simulink model "uas_sim"  (R2020b)
settings: Solver=VariableStepAuto  StartTime=0.0  StopTime=10.0  RelTol=1e-3  SampleTimeConstraint=STIndependent
values from neighbouring files (symbols this model uses):
  framePeriod_s = 1/frameRate_hz    (= 0.02)    [autocode_setup.m]
undefined symbols (not defined in the file or in its folder): Aircraft, datetime, datevec, Earth, Env, InitCond, Telem, WGS84
libraries: aerolibconvert2 x8, simulink x8, aerolibadyn x3, aerolibasang x3, aerolibtransform2 x2, aerolibgravity2 x2, aerolibatmos2 x1, sharedutil x1, aerolibbdyn x1, shared6dof x1
(part 2 of 2)

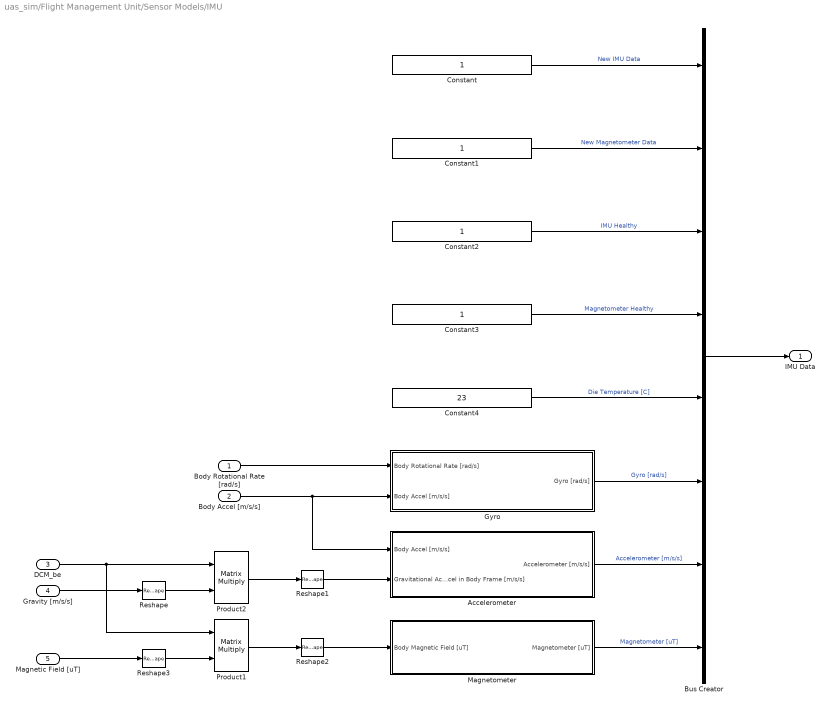
== system uas_sim/Flight Management Unit/Sensor Models/IMU ==
  Body Rotational Rate [rad/s] : Inport
  Body Accel [m/s/s] : Inport  Port=2
  DCM_be : Inport  Port=3
  Gravity [m/s/s] : Inport  Port=4
  Magnetic Field [uT] : Inport  Port=5
  Accelerometer : Subsystem
  Bus Creator : BusCreator  Inputs=8
  Constant{,1..3} (4 alike) : Constant
  Constant4 : Constant  Value=23
  Gyro : Subsystem
  Magnetometer : Subsystem
  Product1 : Product  Multiplication=Matrix(*)
  Product2 : Product  Multiplication=Matrix(*)
  Reshape : Reshape  OutputDimensionality=Column vector (2-D)
  Reshape1 : Reshape
  Reshape2 : Reshape
  Reshape3 : Reshape  OutputDimensionality=Column vector (2-D)
  IMU Data : Outport
  wires:
  Body Accel [m/s/s]/1 -> Accelerometer/1(Body Accel [m/s/s]), Gyro/2(Body Accel [m/s/s])
  DCM_be/1 -> Product2/1, Product1/1
  Gravity [m/s/s]/1 -> Reshape/1
  Bus Creator/1 -> IMU Data/1
  Product2/1 -> Reshape1/1
  Reshape1/1 -> Accelerometer/2(Gravitational Accel in Body Frame [m/s/s])
  Body Rotational Rate [rad/s]/1 -> Gyro/1(Body Rotational Rate [rad/s])
  Reshape2/1 -> Magnetometer/1(Body Magnetic Field [uT])
  Product1/1 -> Reshape2/1
  Reshape3/1 -> Product1/2
  Magnetic Field [uT]/1 -> Reshape3/1
  Magnetometer/1(Magnetometer [uT]) -> Bus Creator/8  "Magnetometer [uT]"
  Accelerometer/1(Accelerometer [m/s/s]) -> Bus Creator/7  "Accelerometer [m/s/s]"
  Gyro/1(Gyro [rad/s]) -> Bus Creator/6  "Gyro [rad/s]"
  Reshape/1 -> Product2/2
  Constant1/1 -> Bus Creator/2  "New Magnetometer Data"
  Constant/1 -> Bus Creator/1  "New IMU Data"
  Constant2/1 -> Bus Creator/3  "IMU Healthy"
  Constant3/1 -> Bus Creator/4  "Magnetometer Healthy"
  Constant4/1 -> Bus Creator/5  "Die Temperature [C]"

== system uas_sim/Flight Management Unit/Sensor Models/Static Pressure Sensor ==
  Pressure : Inport
  Add : Sum  Inputs=+++
  Band-Limited White Noise : simulink/Sources/Band-Limited White Noise  Cov=Aircraft.Sensors.StaticPres.noise_pa  Ts=0.1  seed=[23341]
  Bus Creator : BusCreator  Inputs=4
  Constant : Constant  Value=Aircraft.Sensors.StaticPres.bias_pa
  Constant1 : Constant  Value=Aircraft.Sensors.StaticPres.scale_factor
  Constant2 : Constant  Value=23
  Constant3 : Constant
  Constant4 : Constant
  Product : Product
  Saturation : Saturate  UpperLimit=Aircraft.Sensors.StaticPres.upper_limit_pa  LowerLimit=Aircraft.Sensors.StaticPres.lower_limit_pa
  Pressure Data : Outport
  wires:
  Constant4/1 -> Bus Creator/1  "New Data"
  Constant3/1 -> Bus Creator/2  "Healthy"
  Constant2/1 -> Bus Creator/4  "Die Temperature [C]"
  Saturation/1 -> Bus Creator/3  "Pressure [Pa]"
  Band-Limited White Noise/1 -> Add/1
  Constant/1 -> Add/2
  Add/1 -> Saturation/1
  Product/1 -> Add/3
  Pressure/1 -> Product/1
  Constant1/1 -> Product/2
  Bus Creator/1 -> Pressure Data/1

== system uas_sim/Vehicle/Forces and Moments/Aerodynamic ==
  note: C6 = [CD, CY, CLift, CL, CM, CN]
  Body Velocity [m/s] : Inport
  Body Rotational Rates [rad/s] : Inport  Port=2
  Surface Positions [rad] : Inport  Port=3
  Dynamic Pressure [Pa] : Inport  Port=4
  Angle of Attack [rad] : Inport  Port=5
  Sideslip Angle [rad] : Inport  Port=6
  Airspeed [m/s] : Inport  Port=7
  Add : Sum  Inputs=+++
  Aerodynamic Forces and Moments Coef Axis Variant : Subsystem  Variant=on
  Base Airframe : Subsystem
  Control Derivatives : Subsystem
  Dynamic Derivatives : Subsystem
  Fxyz Mxzy : Outport
  wires:
  Base Airframe/1(C6) -> Add/1
  Dynamic Derivatives/1(dC6) -> Add/2
  Sideslip Angle [rad]/1 -> Base Airframe/2(Sideslip Angle [rad])
  Angle of Attack [rad]/1 -> Base Airframe/1(Angle of Attack [rad]), Control Derivatives/2(Angle of Attack [rad]), Dynamic Derivatives/3(Angle of Attack [rad])
  Body Rotational Rates [rad/s]/1 -> Dynamic Derivatives/2(Body Rotational Rate [rad/s])
  Airspeed [m/s]/1 -> Dynamic Derivatives/1(Airspeed [m/s])
  Surface Positions [rad]/1 -> Control Derivatives/1(Surface Positions [rad])
  Control Derivatives/1(dC6) -> Add/3
  Add/1 -> Aerodynamic Forces and Moments Coef Axis Variant/1(Coef)
  Body Velocity [m/s]/1 -> Aerodynamic Forces and Moments Coef Axis Variant/3(Body Velocity [m/s])
  Dynamic Pressure [Pa]/1 -> Aerodynamic Forces and Moments Coef Axis Variant/2(Dynamic Pressure [Pa])
  Aerodynamic Forces and Moments Coef Axis Variant/1(Fxyz Mxyz) -> Fxyz Mxzy/1

== system uas_sim/Vehicle/Forces and Moments/Gravitational ==
  Gravity [m/s/s] : Inport
  DCM_be : Inport  Port=2
  Gravity Moment : Constant  Value=[0 0 0]
  Mux : Mux  Inputs=2
  Product : Product
  Product1 : Product  Multiplication=Matrix(*)
  Reshape : Reshape  OutputDimensionality=Column vector (2-D)
  Reshape1 : Reshape
  UAV Mass : Constant  Value=Aircraft.Mass.mass_kg
  Fxyz Mxyz : Outport
  wires:
  UAV Mass/1 -> Product/2
  Product/1 -> Product1/2  "Gravity Force NED [N]"
  DCM_be/1 -> Product1/1
  Gravity Moment/1 -> Mux/2
  Mux/1 -> Fxyz Mxyz/1
  Reshape/1 -> Product/1
  Gravity [m/s/s]/1 -> Reshape/1
  Reshape1/1 -> Mux/1
  Product1/1 -> Reshape1/1  "Gravity Force Body [N]"

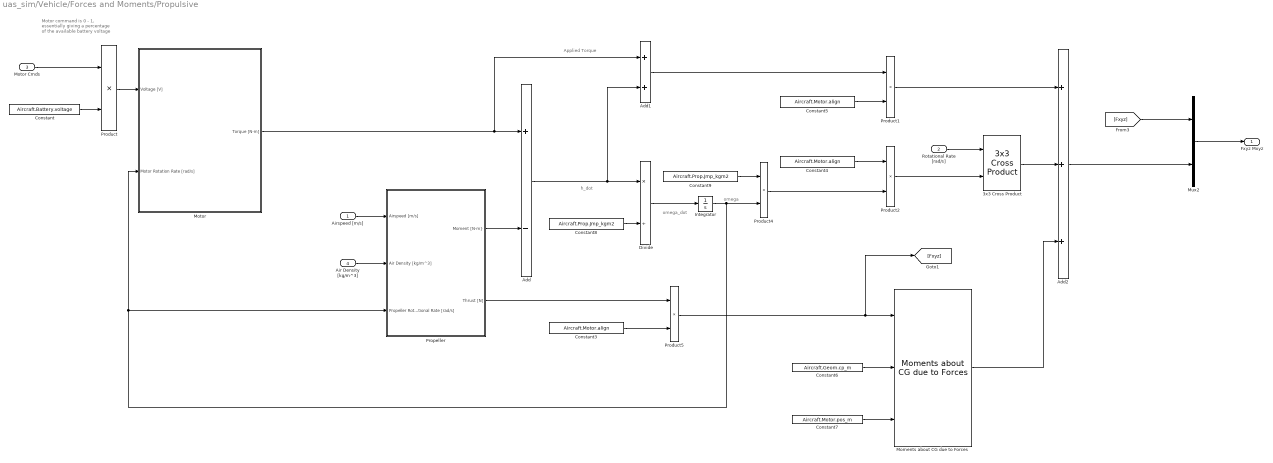
== system uas_sim/Vehicle/Forces and Moments/Propulsive ==
  note: Applied Torque
  note: omega_dot
  note: Motor command is 0 - 1,
      | essentially giving a percentage
      | of the available battery voltage
  note: h_dot
  note: omega
  Airspeed [m/s] : Inport
  Rotational Rate [rad/s] : Inport  Port=2
  Motor Cmds : Inport  Port=3
  Air Density [kg/m^3] : Inport  Port=4
  3x3 Cross Product : sharedutil/3x3 Cross Product  aMode=aMode
      settings: SourceProductBaseCode=AE,PW,MT,UV,VE,VP
  Add : Sum  Inputs=+-
  Add1 : Sum
  Add2 : Sum  Inputs=+++
  Constant : Constant  Value=Aircraft.Battery.voltage
  Constant3 : Constant  Value=Aircraft.Motor.align
  Constant4 : Constant  Value=Aircraft.Motor.align
  Constant5 : Constant  Value=Aircraft.Motor.align
  Constant6 : Constant  Value=Aircraft.Geom.cp_m
  Constant7 : Constant  Value=Aircraft.Motor.pos_m
  Constant8 : Constant  Value=Aircraft.Prop.Jmp_kgm2
  Constant9 : Constant  Value=Aircraft.Prop.Jmp_kgm2
  Divide : Product  Inputs=*/
  Integrator : Integrator  InitialCondition=InitCond.engine_speed_radps  LowerSaturationLimit=1
  Moments about CG due to Forces : aerolibbdyn/Moments about CG  due to Forces
      settings: SourceProductBaseCode=AE
  Motor : Subsystem
  Mux2 : Mux  Inputs=2
  Product{,1..2,4..5} (5 alike) : Product
  Propeller : Subsystem
  Fxyz Mxyz : Outport
  wires:
  Integrator/1 -> Product4/2, Propeller/3(Propeller Rotational Rate [rad/s]), Motor/2(Motor Rotation Rate [rad/s])
  [Fxyz] -> Mux2/1
  Constant4/1 -> Product2/1
  Motor/1(Torque [N-m]) -> Add1/1, Add/1
  Add1/1 -> Product1/1
  Product/1 -> Motor/1(Voltage [V])
  Moments about CG due to Forces/1 -> Add2/3
  Product1/1 -> Add2/1
  Add2/1 -> Mux2/2
  Constant9/1 -> Product4/1
  Propeller/2(Thrust [N]) -> Product5/1
  3x3 Cross Product/1 -> Add2/2
  Mux2/1 -> Fxyz Mxyz/1
  Constant/1 -> Product/2
  Product5/1 -> [Fxyz], Moments about CG due to Forces/1
  Constant3/1 -> Product5/2
  Divide/1 -> Integrator/1
  Add/1 -> Add1/2, Divide/1
  Propeller/1("Moment [N-m}") -> Add/2
  Constant6/1 -> Moments about CG due to Forces/2
  Rotational Rate [rad/s]/1 -> 3x3 Cross Product/1
  Air Density [kg/m^3]/1 -> Propeller/2(Air Density [kg/m^3])
  Product4/1 -> Product2/2
  Constant7/1 -> Moments about CG due to Forces/3
  Constant8/1 -> Divide/2
  Product2/1 -> 3x3 Cross Product/2
  Constant5/1 -> Product1/2
  Motor Cmds/1 -> Product/1
  Airspeed [m/s]/1 -> Propeller/1(Airspeed [m/s])

== system uas_sim/Vehicle/Vehicle Model/Norm ==
  2D Vector : Inport
  Product : Product
  Sqrt : Sqrt  SaturateOnIntegerOverflow=on
  Sum of Elements : Sum  Inputs=+
  Norm : Outport
  wires:
  2D Vector/1 -> Product/2, Product/1
  Product/1 -> Sum of Elements/1
  Sum of Elements/1 -> Sqrt/1
  Sqrt/1 -> Norm/1

== system uas_sim/Flight Management Unit/Control Laws/Virtual to Non-Virtual Mapping1/Virtual to Non-Virtual Mapping1 ==
  Virtual : Inport
  Bus Creator : BusCreator  Inputs=10
  Bus Selector : BusSelector  OutputSignals=New Data,Lost Frame,Failsafe,Throttle Enable,Mode 0,Mode 1,Throttle,Pitch,Roll,Yaw
  Data Type Conversion{,1..3} (4 alike) : DataTypeConversion  OutDataTypeStr=boolean
  Data Type Conversion4 : DataTypeConversion  OutDataTypeStr=int8
  Data Type Conversion5 : DataTypeConversion  OutDataTypeStr=int8
  Data Type Conversion{6..9} (4 alike) : DataTypeConversion  OutDataTypeStr=single
  Non-Virtual : Outport  OutDataTypeStr=Bus: InceptorData
  wires:
  Virtual/1 -> Bus Selector/1
  Bus Creator/1 -> Non-Virtual/1
  Bus Selector/1 -> Data Type Conversion/1  "<New Data>"
  Data Type Conversion/1 -> Bus Creator/1  "new_data"
  Bus Selector/2 -> Data Type Conversion1/1  "<Lost Frame>"
  Bus Selector/3 -> Data Type Conversion2/1  "<Failsafe>"
  Bus Selector/4 -> Data Type Conversion3/1  "<Throttle Enable>"
  Bus Selector/5 -> Data Type Conversion4/1  "<Mode 0>"
  Bus Selector/6 -> Data Type Conversion5/1  "<Mode 1>"
  Bus Selector/7 -> Data Type Conversion6/1  "<Throttle>"
  Bus Selector/8 -> Data Type Conversion7/1  "<Pitch>"
  Bus Selector/9 -> Data Type Conversion8/1  "<Roll>"
  Bus Selector/10 -> Data Type Conversion9/1  "<Yaw>"
  Data Type Conversion1/1 -> Bus Creator/2  "lost_frame"
  Data Type Conversion2/1 -> Bus Creator/3  "failsafe"
  Data Type Conversion3/1 -> Bus Creator/4  "throttle_en"
  Data Type Conversion4/1 -> Bus Creator/5  "mode0"
  Data Type Conversion5/1 -> Bus Creator/6  "mode1"
  Data Type Conversion6/1 -> Bus Creator/7  "throttle"
  Data Type Conversion7/1 -> Bus Creator/8  "pitch"
  Data Type Conversion8/1 -> Bus Creator/9  "roll"
  Data Type Conversion9/1 -> Bus Creator/10  "yaw"

== system uas_sim/Flight Management Unit/Control Laws/Virtual to Non-Virtual Mapping1/Virtual to Non-Virtual Mapping2 ==
  Virtual : Inport
  Bus Creator : BusCreator  Inputs=8
  Bus Selector : BusSelector  OutputSignals=New IMU Data,New Magnetometer Data,IMU Healthy,Magnetometer Healthy,Die Temperature [C],Accelerometer [m/s/s],Gyro [rad/s],Magnetometer [uT]
  Data Type Conversion{,1..3} (4 alike) : DataTypeConversion  OutDataTypeStr=boolean
  Data Type Conversion{4..7} (4 alike) : DataTypeConversion  OutDataTypeStr=single
  Non-Virtual : Outport  OutDataTypeStr=Bus: ImuData
  wires:
  Bus Creator/1 -> Non-Virtual/1
  Virtual/1 -> Bus Selector/1
  Bus Selector/1 -> Data Type Conversion/1  "<New IMU Data>"
  Data Type Conversion/1 -> Bus Creator/1  "new_imu_data"
  Bus Selector/2 -> Data Type Conversion1/1  "<New Magnetometer Data>"
  Data Type Conversion1/1 -> Bus Creator/2  "new_mag_data"
  Bus Selector/3 -> Data Type Conversion2/1  "<IMU Healthy>"
  Data Type Conversion2/1 -> Bus Creator/3  "imu_healthy"
  Bus Selector/4 -> Data Type Conversion3/1  "<Magnetometer Healthy>"
  Data Type Conversion3/1 -> Bus Creator/4  "mag_healthy"
  Bus Selector/5 -> Data Type Conversion4/1  "<Die Temperature [C]>"
  Data Type Conversion4/1 -> Bus Creator/5  "die_temp_c"
  Bus Selector/6 -> Data Type Conversion5/1  "<Accelerometer [m/s/s]>"
  Bus Selector/7 -> Data Type Conversion6/1  "<Gyro [rad/s]>"
  Bus Selector/8 -> Data Type Conversion7/1  "<Magnetometer [uT]>"
  Data Type Conversion5/1 -> Bus Creator/6  "accel_mps2"
  Data Type Conversion6/1 -> Bus Creator/7  "gyro_radps"
  Data Type Conversion7/1 -> Bus Creator/8  "mag_ut"

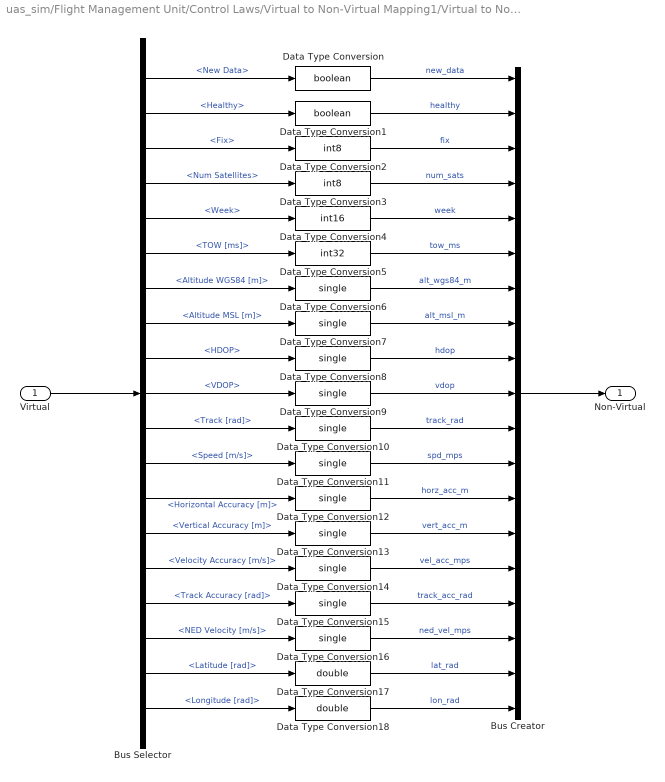
== system uas_sim/Flight Management Unit/Control Laws/Virtual to Non-Virtual Mapping1/Virtual to Non-Virtual Mapping3 ==
  Virtual : Inport
  Bus Creator : BusCreator  Inputs=19
  Bus Selector : BusSelector  OutputSignals=New Data,Healthy,Fix,Num Satellites,Week,TOW [ms],Altitude WGS84 [m],Altitude MSL [m],HDOP,VDOP,Track [rad],Speed [m/s],Horizontal Accuracy [m],Vertical Accuracy [m],Velocity Accuracy [m/s],Track Accuracy [rad],NED Velocity [m/s],Latitude [rad],Longitude [rad]
  Data Type Conversion : DataTypeConversion  OutDataTypeStr=boolean
  Data Type Conversion1 : DataTypeConversion  OutDataTypeStr=boolean
  Data Type Conversion{6..16} (11 alike) : DataTypeConversion  OutDataTypeStr=single
  Data Type Conversion17 : DataTypeConversion  OutDataTypeStr=double
  Data Type Conversion18 : DataTypeConversion  OutDataTypeStr=double
  Data Type Conversion2 : DataTypeConversion  OutDataTypeStr=int8
  Data Type Conversion3 : DataTypeConversion  OutDataTypeStr=int8
  Data Type Conversion4 : DataTypeConversion  OutDataTypeStr=int16
  Data Type Conversion5 : DataTypeConversion  OutDataTypeStr=int32
  Non-Virtual : Outport  OutDataTypeStr=Bus: GnssData
  wires:
  Virtual/1 -> Bus Selector/1
  Bus Creator/1 -> Non-Virtual/1
  Bus Selector/1 -> Data Type Conversion/1  "<New Data>"
  Data Type Conversion/1 -> Bus Creator/1  "new_data"
  Bus Selector/2 -> Data Type Conversion1/1  "<Healthy>"
  Data Type Conversion1/1 -> Bus Creator/2  "healthy"
  Bus Selector/3 -> Data Type Conversion2/1  "<Fix>"
  Data Type Conversion2/1 -> Bus Creator/3  "fix"
  Bus Selector/4 -> Data Type Conversion3/1  "<Num Satellites>"
  Data Type Conversion3/1 -> Bus Creator/4  "num_sats"
  Bus Selector/5 -> Data Type Conversion4/1  "<Week>"
  Data Type Conversion4/1 -> Bus Creator/5  "week"
  Bus Selector/6 -> Data Type Conversion5/1  "<TOW [ms]>"
  Data Type Conversion5/1 -> Bus Creator/6  "tow_ms"
  Bus Selector/7 -> Data Type Conversion6/1  "<Altitude WGS84 [m]>"
  Bus Selector/8 -> Data Type Conversion7/1  "<Altitude MSL [m]>"
  Data Type Conversion6/1 -> Bus Creator/7  "alt_wgs84_m"
  Data Type Conversion7/1 -> Bus Creator/8  "alt_msl_m"
  Bus Selector/9 -> Data Type Conversion8/1  "<HDOP>"
  Bus Selector/10 -> Data Type Conversion9/1  "<VDOP>"
  Data Type Conversion8/1 -> Bus Creator/9  "hdop"
  Data Type Conversion9/1 -> Bus Creator/10  "vdop"
  Bus Selector/11 -> Data Type Conversion10/1  "<Track [rad]>"
  Bus Selector/12 -> Data Type Conversion11/1  "<Speed [m/s]>"
  Data Type Conversion10/1 -> Bus Creator/11  "track_rad"
  Data Type Conversion11/1 -> Bus Creator/12  "spd_mps"
  Bus Selector/13 -> Data Type Conversion12/1  "<Horizontal Accuracy [m]>"
  Bus Selector/14 -> Data Type Conversion13/1  "<Vertical Accuracy [m]>"
  Bus Selector/15 -> Data Type Conversion14/1  "<Velocity Accuracy [m/s]>"
  Bus Selector/16 -> Data Type Conversion15/1  "<Track Accuracy [rad]>"
  Bus Selector/17 -> Data Type Conversion16/1  "<NED Velocity [m/s]>"
  Bus Selector/18 -> Data Type Conversion17/1  "<Latitude [rad]>"
  Bus Selector/19 -> Data Type Conversion18/1  "<Longitude [rad]>"
  Data Type Conversion18/1 -> Bus Creator/19  "lon_rad"
  Data Type Conversion17/1 -> Bus Creator/18  "lat_rad"
  Data Type Conversion16/1 -> Bus Creator/17  "ned_vel_mps"
  Data Type Conversion15/1 -> Bus Creator/16  "track_acc_rad"
  Data Type Conversion14/1 -> Bus Creator/15  "vel_acc_mps"
  Data Type Conversion13/1 -> Bus Creator/14  "vert_acc_m"
  Data Type Conversion12/1 -> Bus Creator/13  "horz_acc_m"

== system uas_sim/Flight Management Unit/Control Laws/Virtual to Non-Virtual Mapping1/Virtual to Non-Virtual Mapping4 ==
  Virtual : Inport
  Bus Creator : BusCreator  Inputs=4
  Bus Selector : BusSelector  OutputSignals=New Data,Healthy,Pressure [Pa],Die Temperature [C]
  Data Type Conversion : DataTypeConversion  OutDataTypeStr=boolean
  Data Type Conversion1 : DataTypeConversion  OutDataTypeStr=boolean
  Data Type Conversion2 : DataTypeConversion  OutDataTypeStr=single
  Data Type Conversion3 : DataTypeConversion  OutDataTypeStr=single
  Non-Virtual : Outport  OutDataTypeStr=Bus: PresData
  wires:
  Bus Creator/1 -> Non-Virtual/1
  Virtual/1 -> Bus Selector/1
  Bus Selector/1 -> Data Type Conversion/1  "<New Data>"
  Data Type Conversion/1 -> Bus Creator/1  "new_data"
  Bus Selector/2 -> Data Type Conversion1/1  "<Healthy>"
  Data Type Conversion1/1 -> Bus Creator/2  "healthy"
  Bus Selector/3 -> Data Type Conversion2/1  "<Pressure [Pa]>"
  Data Type Conversion2/1 -> Bus Creator/3  "pres_pa"
  Bus Selector/4 -> Data Type Conversion3/1  "<Die Temperature [C]>"
  Data Type Conversion3/1 -> Bus Creator/4  "die_temp_c"

== system uas_sim/Flight Management Unit/Control Laws/Virtual to Non-Virtual Mapping1/Virtual to Non-Virtual Mapping5 ==
  Virtual : Inport
  Bus Creator : BusCreator  Inputs=4
  Bus Selector : BusSelector  OutputSignals=New Data,Healthy,Pressure [Pa],Die Temperature [C]
  Data Type Conversion : DataTypeConversion  OutDataTypeStr=boolean
  Data Type Conversion1 : DataTypeConversion  OutDataTypeStr=boolean
  Data Type Conversion2 : DataTypeConversion  OutDataTypeStr=single
  Data Type Conversion3 : DataTypeConversion  OutDataTypeStr=single
  Non-Virtual : Outport  OutDataTypeStr=Bus: PresData
  wires:
  Data Type Conversion3/1 -> Bus Creator/4  "die_temp_c"
  Bus Selector/4 -> Data Type Conversion3/1  "<Die Temperature [C]>"
  Data Type Conversion2/1 -> Bus Creator/3  "pres_pa"
  Bus Selector/3 -> Data Type Conversion2/1  "<Pressure [Pa]>"
  Data Type Conversion1/1 -> Bus Creator/2  "healthy"
  Bus Selector/2 -> Data Type Conversion1/1  "<Healthy>"
  Data Type Conversion/1 -> Bus Creator/1  "new_data"
  Bus Selector/1 -> Data Type Conversion/1  "<New Data>"
  Virtual/1 -> Bus Selector/1
  Bus Creator/1 -> Non-Virtual/1

== system uas_sim/Flight Management Unit/Control Laws/Virtual to Non-Virtual Mapping1/Virtual to Non-Virtual Mapping6 ==
  Virtual : Inport
  Bus Creator : BusCreator  Inputs=2
  Bus Selector : BusSelector  OutputSignals=Voltages,Values
  Data Type Conversion2 : DataTypeConversion  OutDataTypeStr=single
  Data Type Conversion3 : DataTypeConversion  OutDataTypeStr=single
  Non-Virtual : Outport  OutDataTypeStr=Bus: AnalogData
  wires:
  Bus Creator/1 -> Non-Virtual/1
  Virtual/1 -> Bus Selector/1
  Data Type Conversion2/1 -> Bus Creator/1  "volt"
  Bus Selector/1 -> Data Type Conversion2/1  "<Voltages>"
  Bus Selector/2 -> Data Type Conversion3/1  "<Values>"
  Data Type Conversion3/1 -> Bus Creator/2  "val"

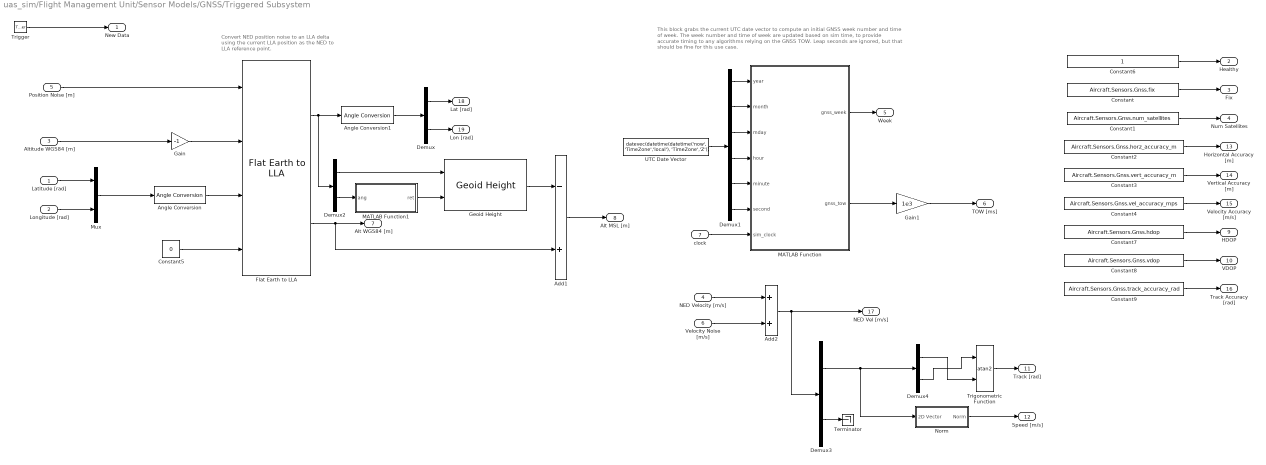
== system uas_sim/Flight Management Unit/Sensor Models/GNSS/Triggered Subsystem ==
  note: This block grabs the current UTC date vector to compute an initial GNSS week number
      | and time of week. The week number and time of week are updated based on sim time, to provide accurate timing to any algorithms relying on the GNSS TOW. Leap seconds are ignored, but that should be fine for this use case.
  note: Convert NED position noise to an LLA delta
      | using the current LLA position as the NED to
      | LLA reference point.
  Latitude [rad] : Inport
  "Longitude [rad] " : Inport  Port=2
  Altitude WGS84 [m] : Inport  Port=3
  NED Velocity [m/s] : Inport  Port=4  PortDimensions=3
  Position Noise [m] : Inport  Port=5  PortDimensions=3
  Velocity Noise [m/s] : Inport  Port=6  PortDimensions=3
  clock : Inport  Port=7
  Trigger : TriggerPort  VariantControl=Variant  ShowOutputPort=on
  Add1 : Sum  Inputs=-+
  Add2 : Sum
  Angle Conversion : aerolibconvert2/Angle Conversion  IU=rad  OU=deg
  Angle Conversion1 : aerolibconvert2/Angle Conversion  IU=deg  OU=rad
  Constant : Constant  Value=Aircraft.Sensors.Gnss.fix
  Constant1 : Constant  Value=Aircraft.Sensors.Gnss.num_satellites
  Constant2 : Constant  Value=Aircraft.Sensors.Gnss.horz_accuracy_m
  Constant3 : Constant  Value=Aircraft.Sensors.Gnss.vert_accuracy_m
  Constant4 : Constant  Value=Aircraft.Sensors.Gnss.vel_accuracy_mps
  Constant5 : Constant  Value=0
  Constant6 : Constant
  Constant7 : Constant  Value=Aircraft.Sensors.Gnss.hdop
  Constant8 : Constant  Value=Aircraft.Sensors.Gnss.vdop
  Constant9 : Constant  Value=Aircraft.Sensors.Gnss.track_accuracy_rad
  Demux : Demux  Outputs=2
  Demux1 : Demux  Outputs=6
  Demux2 : Demux  Outputs=2
  Demux3 : Demux  Outputs=[2 1]
  Demux4 : Demux  Outputs=2
  Flat Earth to LLA : aerolibtransform2/Flat Earth to LLA  units=Metric (MKS)  ptype=Earth (WGS84)  F=1/298.257223563  R=6378137  refPosPort=on  LL0=[0 10]  psi=0
  Gain : Gain  Gain=-1
  Gain1 : Gain  Gain=1e3
  Geoid Height : aerolibgravity2/Geoid Height  units=Metric (MKS)  gtype=EGM96  datafile='geoidegm96grid'  dtype=double  action=Warning
      settings: SourceProductBaseCode=AE
  MATLAB Function : MATLAB Function  TreatAsAtomicUnit=on
  MATLAB Function1 : MATLAB Function  TreatAsAtomicUnit=on
  Mux : Mux  Inputs=2
  Norm : Subsystem
  Terminator : Terminator
  Trigonometric Function : Trigonometry  Operator=atan2
  UTC Date Vector : Constant  Value=datevec(datetime(datetime('now', 'TimeZone','local'), 'TimeZone','Z'))  SampleTime=-1
  New Data : Outport
  Healthy : Outport  Port=2
  Fix : Outport  Port=3
  Num Satellites : Outport  Port=4
  Week : Outport  Port=5
  TOW [ms] : Outport  Port=6
  Alt WGS84 [m] : Outport  Port=7
  Alt MSL [m] : Outport  Port=8
  HDOP : Outport  Port=9
  VDOP : Outport  Port=10
  Track [rad] : Outport  Port=11
  Speed [m/s] : Outport  Port=12
  Horizontal Accuracy [m] : Outport  Port=13
  Vertical Accuracy [m] : Outport  Port=14
  Velocity Accuracy [m/s] : Outport  Port=15
  Track Accuracy [rad] : Outport  Port=16
  NED Vel [m/s] : Outport  Port=17
  Lat [rad] : Outport  Port=18
  Lon [rad] : Outport  Port=19
  wires:
  Constant/1 -> Fix/1
  Constant1/1 -> Num Satellites/1
  Constant2/1 -> Horizontal Accuracy [m]/1
  Constant3/1 -> Vertical Accuracy [m]/1
  Constant4/1 -> Velocity Accuracy [m/s]/1
  Position Noise [m]/1 -> Flat Earth to LLA/1
  Altitude WGS84 [m]/1 -> Gain/1
  Mux/1 -> Angle Conversion/1
  Angle Conversion/1 -> Flat Earth to LLA/3
  Constant5/1 -> Flat Earth to LLA/4
  "Longitude [rad] "/1 -> Mux/2
  Latitude [rad]/1 -> Mux/1
  Flat Earth to LLA/1 -> Demux2/1, Angle Conversion1/1
  Angle Conversion1/1 -> Demux/1
  Demux/2 -> Lon [rad]/1
  Demux/1 -> Lat [rad]/1
  Flat Earth to LLA/2 -> Add1/2, Alt WGS84 [m]/1
  NED Velocity [m/s]/1 -> Add2/1
  Add2/1 -> Demux3/1, NED Vel [m/s]/1
  Demux1/2 -> MATLAB Function/2(month)
  Demux1/6 -> MATLAB Function/6(second)
  UTC Date Vector/1 -> Demux1/1
  Demux1/1 -> MATLAB Function/1(year)
  Demux1/5 -> MATLAB Function/5(minute)
  Demux1/4 -> MATLAB Function/4(hour)
  Demux1/3 -> MATLAB Function/3(mday)
  MATLAB Function/2(gnss_tow) -> Gain1/1
  MATLAB Function/1(gnss_week) -> Week/1
  clock/1 -> MATLAB Function/7(sim_clock)
  Gain/1 -> Flat Earth to LLA/2
  Constant6/1 -> Healthy/1
  Trigger/1 -> New Data/1
  Gain1/1 -> TOW [ms]/1
  Demux2/1 -> Geoid Height/1
  Demux2/2 -> MATLAB Function1/1(ang)
  MATLAB Function1/1(ret) -> Geoid Height/2
  Geoid Height/1 -> Add1/1
  Add1/1 -> Alt MSL [m]/1
  Constant7/1 -> HDOP/1
  Constant8/1 -> VDOP/1
  Demux4/1 -> Trigonometric Function/2
  Demux4/2 -> Trigonometric Function/1
  Trigonometric Function/1 -> Track [rad]/1
  Velocity Noise [m/s]/1 -> Add2/2
  Constant9/1 -> Track Accuracy [rad]/1
  Demux3/1 -> Norm/1(2D Vector), Demux4/1
  Demux3/2 -> Terminator/1
  Norm/1(Norm) -> Speed [m/s]/1

== system uas_sim/Flight Management Unit/Sensor Models/IMU/Accelerometer ==
  Body Accel [m/s/s] : Inport  PortDimensions=3
  Gravitational Accel in Body Frame [m/s/s] : Inport  Port=2  PortDimensions=3
  Add : Sum  Inputs=+++
  Band-Limited White Noise : simulink/Sources/Band-Limited White Noise  Cov=Aircraft.Sensors.Imu.Accel.noise_mps2  Ts=0.1  seed=[23341]
  Constant : Constant  Value=Aircraft.Sensors.Imu.Accel.bias_mps2  VectorParams1D=off
  Constant1 : Constant  Value=Aircraft.Sensors.Imu.Accel.scale_factor
  Product : Product  Multiplication=Matrix(*)
  Reshape : Reshape  OutputDimensionality=Column vector (2-D)
  Reshape1 : Reshape  OutputDimensionality=Column vector (2-D)
  Reshape2 : Reshape
  Saturation : Saturate  UpperLimit=Aircraft.Sensors.Imu.Accel.upper_limit_mps2  LowerLimit=Aircraft.Sensors.Imu.Accel.lower_limit_mps2
  Subtract : Sum  Inputs=+-
  Accelerometer [m/s/s] : Outport  PortDimensions=3
  wires:
  Add/1 -> Saturation/1
  Band-Limited White Noise/1 -> Add/1
  Product/1 -> Add/3
  Constant/1 -> Add/2
  Constant1/1 -> Product/1
  Subtract/1 -> Product/2
  Reshape/1 -> Subtract/2
  Gravitational Accel in Body Frame [m/s/s]/1 -> Reshape/1
  Reshape1/1 -> Subtract/1
  Body Accel [m/s/s]/1 -> Reshape1/1
  Saturation/1 -> Reshape2/1
  Reshape2/1 -> Accelerometer [m/s/s]/1

== system uas_sim/Flight Management Unit/Sensor Models/IMU/Gyro ==
  Body Rotational Rate [rad/s] : Inport  PortDimensions=3
  Body Accel [m/s/s] : Inport  Port=2  PortDimensions=3
  Add1 : Sum  Inputs=++++
  Band-Limited White Noise : simulink/Sources/Band-Limited White Noise  Cov=Aircraft.Sensors.Imu.Gyro.noise_radps  Ts=0.1  seed=[23341]  VectorParams1D=off
  Constant1 : Constant  Value=Aircraft.Sensors.Imu.Gyro.bias_radps  VectorParams1D=off
  Constant2 : Constant  Value=Aircraft.Sensors.Imu.Gyro.accel_sens_radps
  Constant3 : Constant  Value=Aircraft.Sensors.Imu.Gyro.scale_factor  VectorParams1D=off
  Product : Product
  Product1 : Product  Multiplication=Matrix(*)
  Reshape : Reshape  OutputDimensionality=Column vector (2-D)
  Reshape1 : Reshape  OutputDimensionality=Column vector (2-D)
  Reshape2 : Reshape
  Saturation : Saturate  UpperLimit=Aircraft.Sensors.Imu.Gyro.upper_limit_radps  LowerLimit=Aircraft.Sensors.Imu.Gyro.lower_limit_radps
  Gyro [rad/s] : Outport  PortDimensions=3
  wires:
  Constant3/1 -> Product1/1
  Constant2/1 -> Product/1
  Add1/1 -> Saturation/1
  Constant1/1 -> Add1/3
  Product1/1 -> Add1/4
  Band-Limited White Noise/1 -> Add1/2
  Body Rotational Rate [rad/s]/1 -> Reshape/1
  Reshape/1 -> Product1/2
  Body Accel [m/s/s]/1 -> Product/2
  Product/1 -> Reshape1/1
  Reshape1/1 -> Add1/1
  Reshape2/1 -> Gyro [rad/s]/1
  Saturation/1 -> Reshape2/1

== system uas_sim/Flight Management Unit/Sensor Models/IMU/Magnetometer ==
  Body Magnetic Field [uT] : Inport  PortDimensions=3
  Add2 : Sum  Inputs=+++
  Band-Limited White Noise : simulink/Sources/Band-Limited White Noise  Cov=Aircraft.Sensors.Imu.Mag.noise_ut  Ts=0.1  seed=[23341]
  Constant1 : Constant  Value=Aircraft.Sensors.Imu.Mag.scale_factor  VectorParams1D=off
  Constant2 : Constant  Value=Aircraft.Sensors.Imu.Mag.bias_ut
  Product : Product  Multiplication=Matrix(*)
  Reshape : Reshape  OutputDimensionality=Column vector (2-D)
  Reshape1 : Reshape
  Saturation : Saturate  UpperLimit=Aircraft.Sensors.Imu.Mag.upper_limit_ut  LowerLimit=Aircraft.Sensors.Imu.Mag.lower_limit_ut
  Magnetometer [uT] : Outport  PortDimensions=3
  wires:
  Body Magnetic Field [uT]/1 -> Reshape/1
  Band-Limited White Noise/1 -> Add2/1
  Add2/1 -> Saturation/1
  Constant2/1 -> Add2/2
  Constant1/1 -> Product/1
  Reshape/1 -> Product/2
  Saturation/1 -> Reshape1/1
  Reshape1/1 -> Magnetometer [uT]/1
  Product/1 -> Add2/3

== system uas_sim/Vehicle/Forces and Moments/Aerodynamic/Aerodynamic Forces and Moments Coef Axis Variant ==
  Coef : Inport
  Dynamic Pressure [Pa] : Inport  Port=2
  Body Velocity [m/s] : Inport  Port=3
  Body Axis Coef : Subsystem  VariantControl=Aircraft.Aero.axis == 3
  Stability Axis Coef : Subsystem  VariantControl=Aircraft.Aero.axis == 2
  Wind Axis Coef : Subsystem  VariantControl=Aircraft.Aero.axis == 1
  Fxyz Mxyz : Outport

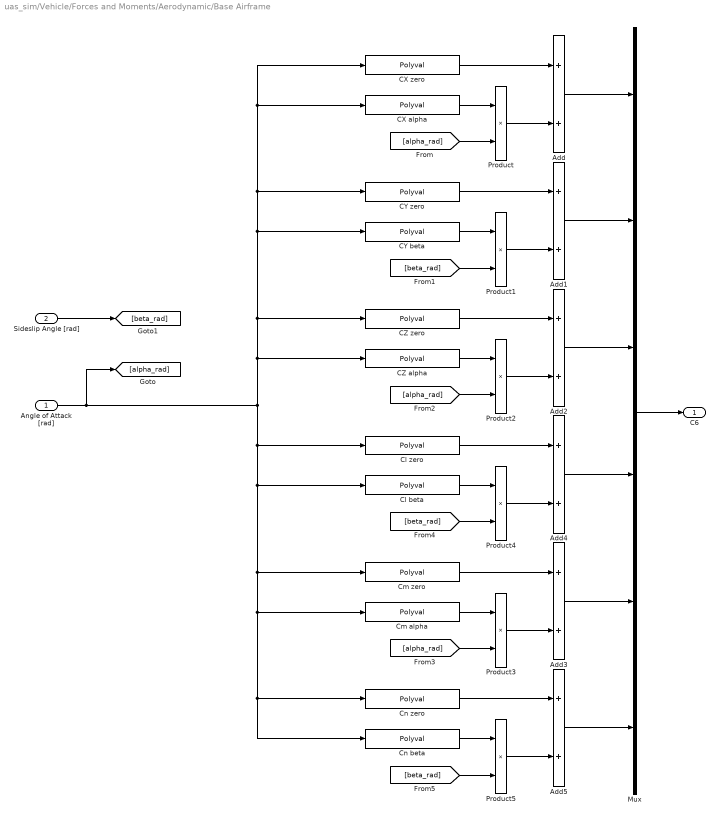
== system uas_sim/Vehicle/Forces and Moments/Aerodynamic/Base Airframe ==
  Angle of Attack [rad] : Inport
  Sideslip Angle [rad] : Inport  Port=2
  Add{,1..5} (6 alike) : Sum
  CX alpha : Polyval  Coefs=Aircraft.Aero.CX.alpha
  CX zero : Polyval  Coefs=Aircraft.Aero.CX.zero
  CY beta : Polyval  Coefs=Aircraft.Aero.CY.beta
  CY zero : Polyval  Coefs=Aircraft.Aero.CY.zero
  CZ alpha : Polyval  Coefs=Aircraft.Aero.CZ.alpha
  CZ zero : Polyval  Coefs=Aircraft.Aero.CZ.zero
  Cl beta : Polyval  Coefs=Aircraft.Aero.Cl.beta
  Cl zero : Polyval  Coefs=Aircraft.Aero.Cl.zero
  Cm alpha : Polyval  Coefs=Aircraft.Aero.Cm.alpha
  Cm zero : Polyval  Coefs=Aircraft.Aero.Cm.zero
  Cn beta : Polyval  Coefs=Aircraft.Aero.Cn.beta
  Cn zero : Polyval  Coefs=Aircraft.Aero.Cn.zero
  Mux : Mux  Inputs=6
  Product{,1..5} (6 alike) : Product
  C6 : Outport
  wires:
  Product/1 -> Add/2
  Add/1 -> Mux/1
  CX alpha/1 -> Product/1
  CX zero/1 -> Add/1
  Sideslip Angle [rad]/1 -> [beta_rad]
  [alpha_rad] -> Product/2
  Mux/1 -> C6/1
  [beta_rad] -> Product1/2
  CY zero/1 -> Add1/1
  CY beta/1 -> Product1/1
  Product1/1 -> Add1/2
  Add1/1 -> Mux/2
  CZ zero/1 -> Add2/1
  CZ alpha/1 -> Product2/1
  Add2/1 -> Mux/3
  Product2/1 -> Add2/2
  Product3/1 -> Add3/2
  Add3/1 -> Mux/5
  Cm alpha/1 -> Product3/1
  Cm zero/1 -> Add3/1
  [alpha_rad] -> Product2/2
  [alpha_rad] -> Product3/2
  Add4/1 -> Mux/4
  Product4/1 -> Add4/2
  Cl beta/1 -> Product4/1
  Cl zero/1 -> Add4/1
  [beta_rad] -> Product4/2
  [beta_rad] -> Product5/2
  Cn zero/1 -> Add5/1
  Cn beta/1 -> Product5/1
  Product5/1 -> Add5/2
  Add5/1 -> Mux/6
  Angle of Attack [rad]/1 -> [alpha_rad], Cl zero/1, Cl beta/1, Cm zero/1, Cm alpha/1, Cn zero/1, Cn beta/1, CZ alpha/1, CZ zero/1, CY beta/1, CY zero/1, CX alpha/1, CX zero/1

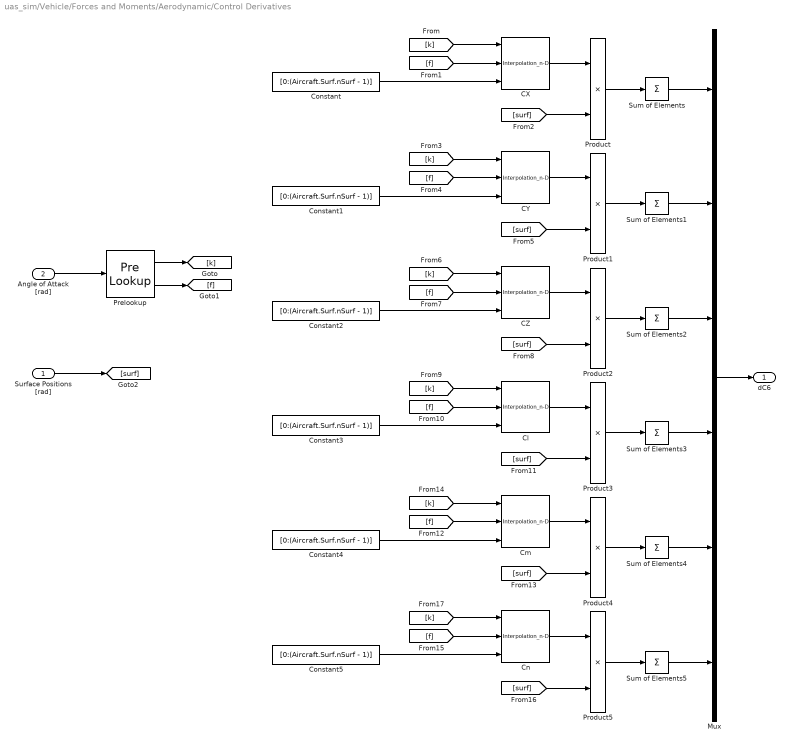
== system uas_sim/Vehicle/Forces and Moments/Aerodynamic/Control Derivatives ==
  Surface Positions [rad] : Inport
  Angle of Attack [rad] : Inport  Port=2
  CX : Interpolation_n-D  Table=Aircraft.Aero.CX.surf  DiagnosticForOutOfRangeInput=Warning  NumSelectionDims=1  InternalRulePriority=Speed
      settings: InputPortMap=u0,u1,u2
  CY : Interpolation_n-D  Table=Aircraft.Aero.CY.surf  DiagnosticForOutOfRangeInput=Warning  NumSelectionDims=1  InternalRulePriority=Speed
      settings: InputPortMap=u0,u1,u2
  CZ : Interpolation_n-D  Table=Aircraft.Aero.CZ.surf  DiagnosticForOutOfRangeInput=Warning  NumSelectionDims=1  InternalRulePriority=Speed
      settings: InputPortMap=u0,u1,u2
  Cl : Interpolation_n-D  Table=Aircraft.Aero.Cl.surf  DiagnosticForOutOfRangeInput=Warning  NumSelectionDims=1  InternalRulePriority=Speed
      settings: InputPortMap=u0,u1,u2
  Cm : Interpolation_n-D  Table=Aircraft.Aero.Cm.surf  DiagnosticForOutOfRangeInput=Warning  NumSelectionDims=1  InternalRulePriority=Speed
      settings: InputPortMap=u0,u1,u2
  Cn : Interpolation_n-D  Table=Aircraft.Aero.Cn.surf  DiagnosticForOutOfRangeInput=Warning  NumSelectionDims=1  InternalRulePriority=Speed
      settings: InputPortMap=u0,u1,u2
  Constant{,1..5} (6 alike) : Constant  Value=[0:(Aircraft.Surf.nSurf - 1)]
  Mux : Mux  Inputs=6
  Prelookup : PreLookup  BreakpointsData=Aircraft.Aero.CntrlEff.alpha  ExtrapMethod=Linear
  Product{,1..5} (6 alike) : Product
  Sum of Elements{,1..5} (6 alike) : Sum  Inputs=+
  dC6 : Outport
  wires:
  [k] -> Cm/1
  CY/1 -> Product1/1
  [f] -> Cn/2
  Product5/1 -> Sum of Elements5/1
  [surf] -> Product5/2
  Constant4/1 -> Cm/3
  Sum of Elements1/1 -> Mux/2
  [k] -> Cn/1
  Sum of Elements5/1 -> Mux/6
  Constant3/1 -> Cl/3
  [surf] -> Product3/2
  [k] -> Cl/1
  [f] -> Cl/2
  Constant2/1 -> CZ/3
  [k] -> CZ/1
  [surf] -> Product2/2
  Cl/1 -> Product3/1
  CZ/1 -> Product2/1
  Product2/1 -> Sum of Elements2/1
  Product3/1 -> Sum of Elements3/1
  Product1/1 -> Sum of Elements1/1
  Product/1 -> Sum of Elements/1
  [k] -> CY/1
  [f] -> CY/2
  Constant1/1 -> CY/3
  Constant/1 -> CX/3
  Cm/1 -> Product4/1
  [k] -> CX/1
  [surf] -> Product/2
  Prelookup/2 -> [f]
  Mux/1 -> dC6/1
  Prelookup/1 -> [k]
  Product4/1 -> Sum of Elements4/1
  Cn/1 -> Product5/1
  Angle of Attack [rad]/1 -> Prelookup/1
  Surface Positions [rad]/1 -> [surf]
  [f] -> CZ/2
  [f] -> Cm/2
  Sum of Elements2/1 -> Mux/3
  CX/1 -> Product/1
  [f] -> CX/2
  Constant5/1 -> Cn/3
  [surf] -> Product4/2
  Sum of Elements/1 -> Mux/1
  Sum of Elements4/1 -> Mux/5
  [surf] -> Product1/2
  Sum of Elements3/1 -> Mux/4

== system uas_sim/Vehicle/Forces and Moments/Aerodynamic/Dynamic Derivatives ==
  note: Divide by zero protection
  Airspeed [m/s] : Inport
  Body Rotational Rate [rad/s] : Inport  Port=2
  Angle of Attack [rad] : Inport  Port=3
  Add : Sum  Inputs=+++
  Constant : Constant  Value=Aircraft.Geom.b_m
  Constant1 : Constant  Value=Aircraft.Geom.c_m
  Constant2 : Constant  Value=Aircraft.Geom.b_m
  Demux : Demux  Outputs=3
  Divide : Product  Inputs=*/
  Gain : Gain  Gain=2
  Mux : Mux  Inputs=3
  Pitch Rate : Subsystem
  Product : Product
  Roll Rate : Subsystem
  Saturation : Saturate  UpperLimit=inf  LowerLimit=1e-3
  Yaw Rate : Subsystem
  dC6 : Outport
  wires:
  Constant/1 -> Mux/1
  Body Rotational Rate [rad/s]/1 -> Product/1
  Mux/1 -> Product/2
  Airspeed [m/s]/1 -> Gain/1
  Gain/1 -> Saturation/1
  Product/1 -> Divide/1
  Saturation/1 -> Divide/2
  Divide/1 -> Demux/1
  Demux/1 -> Roll Rate/2(p_hat)
  Demux/2 -> Pitch Rate/2(q_hat)
  Demux/3 -> Yaw Rate/2(r_hat)
  Angle of Attack [rad]/1 -> Yaw Rate/1(Angle of Attack [rad]), Pitch Rate/1(Angle of Attack [rad]), Roll Rate/1(Angle of Attack [rad])
  Roll Rate/1(dC6) -> Add/1
  Pitch Rate/1(dC6) -> Add/2
  Yaw Rate/1(dC6) -> Add/3
  Constant2/1 -> Mux/3
  Constant1/1 -> Mux/2
  Add/1 -> dC6/1

== system uas_sim/Vehicle/Forces and Moments/Propulsive/Motor ==
  note: RPM to rad/s
  Voltage [V] : Inport
  Motor Rotation Rate [rad/s] : Inport  Port=2
  Constant : Constant  Value=Aircraft.Motor.kv
  Constant1 : Constant  Value=Aircraft.Motor.io
  Divide : Product  Inputs=*/
  Divide2 : Product  Inputs=*/
  Gain : Gain  Gain=1/Aircraft.Motor.r
  Gain2 : Gain  Gain=2 * pi / 60
  Subtract : Sum  Inputs=+-
  Subtract1 : Sum  Inputs=+-
  Torque [N-m] : Outport
  wires:
  Gain2/1 -> [KvSI], Divide/2
  [KvSI] -> Divide2/2
  Constant1/1 -> Subtract1/2
  Motor Rotation Rate [rad/s]/1 -> Divide/1
  Divide/1 -> Subtract/2
  Constant/1 -> Gain2/1
  Gain/1 -> Subtract1/1
  Subtract1/1 -> Divide2/1
  Voltage [V]/1 -> Subtract/1
  Divide2/1 -> Torque [N-m]/1
  Subtract/1 -> Gain/1

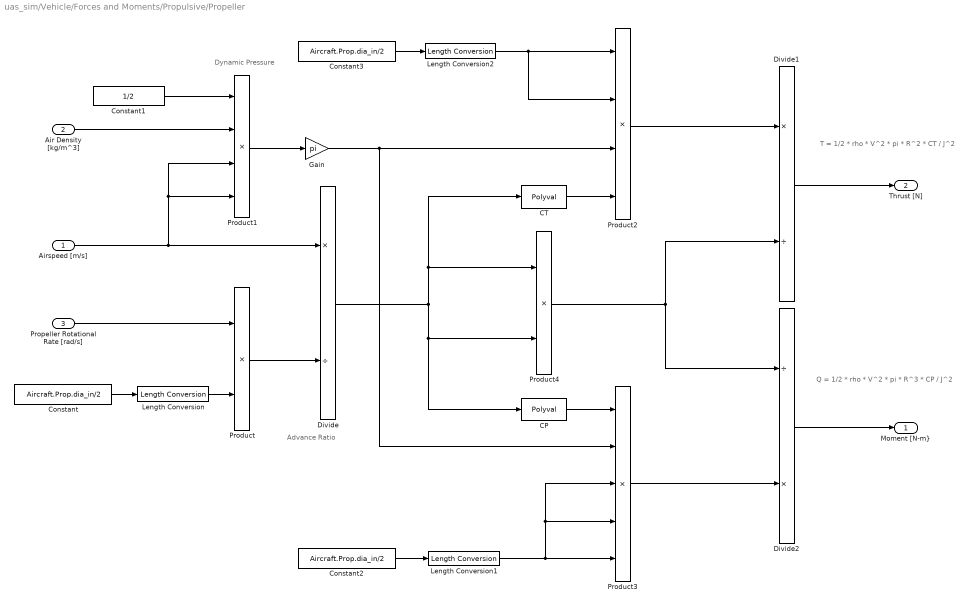
== system uas_sim/Vehicle/Forces and Moments/Propulsive/Propeller ==
  note: Dynamic Pressure
  note: Q = 1/2 * rho * V^2 * pi * R^3 * CP / J^2
  note: T = 1/2 * rho * V^2 * pi * R^2 * CT / J^2
  note: Advance Ratio
  Airspeed [m/s] : Inport
  Air Density [kg/m^3] : Inport  Port=2
  Propeller Rotational Rate [rad/s] : Inport  Port=3
  CP : Polyval  Coefs=Aircraft.prop.cp
  CT : Polyval  Coefs=Aircraft.prop.ct
  Constant : Constant  Value=Aircraft.Prop.dia_in/2
  Constant1 : Constant  Value=1/2
  Constant2 : Constant  Value=Aircraft.Prop.dia_in/2
  Constant3 : Constant  Value=Aircraft.Prop.dia_in/2
  Divide : Product  Inputs=*/
  Divide1 : Product  Inputs=*/
  Divide2 : Product  Inputs=/*
  Gain : Gain  Gain=pi
  Length Conversion : aerolibconvert2/Length Conversion  IU=in  OU=m
  Length Conversion1 : aerolibconvert2/Length Conversion  IU=in  OU=m
  Length Conversion2 : aerolibconvert2/Length Conversion  IU=in  OU=m
  Product : Product
  Product1 : Product  Inputs=4
  Product2 : Product  Inputs=4
  Product3 : Product  Inputs=5
  Product4 : Product
  "Moment [N-m}" : Outport
  Thrust [N] : Outport  Port=2
  wires:
  Divide2/1 -> "Moment [N-m}"/1
  Length Conversion/1 -> Product/2
  Product4/1 -> Divide2/1, Divide1/2
  Constant2/1 -> Length Conversion1/1
  Airspeed [m/s]/1 -> Divide/1, Product1/4, Product1/3
  Propeller Rotational Rate [rad/s]/1 -> Product/1
  Length Conversion1/1 -> Product3/4, Product3/3, Product3/5
  Product1/1 -> Gain/1
  Gain/1 -> Product3/2, Product2/3
  Air Density [kg/m^3]/1 -> Product1/2
  Divide1/1 -> Thrust [N]/1
  Product3/1 -> Divide2/2
  Constant1/1 -> Product1/1
  CP/1 -> Product3/1
  CT/1 -> Product2/4
  Product2/1 -> Divide1/1
  Length Conversion2/1 -> Product2/2, Product2/1
  Constant/1 -> Length Conversion/1
  Constant3/1 -> Length Conversion2/1
  Divide/1 -> Product4/2, CP/1, Product4/1, CT/1
  Product/1 -> Divide/2

== system uas_sim/Flight Management Unit/Sensor Models/GNSS/Triggered Subsystem/Norm ==
  2D Vector : Inport
  Product : Product
  Sqrt : Sqrt  SaturateOnIntegerOverflow=on
  Sum of Elements : Sum  Inputs=+
  Norm : Outport
  wires:
  2D Vector/1 -> Product/2, Product/1
  Product/1 -> Sum of Elements/1
  Sum of Elements/1 -> Sqrt/1
  Sqrt/1 -> Norm/1

== system uas_sim/Vehicle/Forces and Moments/Aerodynamic/Aerodynamic Forces and Moments Coef Axis Variant/Body Axis Coef ==
  Coef : Inport
  Dynamic Pressure [Pa] : Inport  Port=2
  Body Velocity [m/s] : Inport  Port=3
  "Aerodynamic Forces and Moments " : aerolibadyn/Aerodynamic Forces and Moments   inputAxes=Body  outputForceAxes=Body  outputMomentAxes=Body  S=Aircraft.Geom.s_m2  b=Aircraft.Geom.b_m  cbar=Aircraft.Geom.c_m
  Constant : Constant  Value=Aircraft.Mass.cg_m
  Constant1 : Constant  Value=Aircraft.Geom.cp_m
  Mux : Mux  Inputs=2
  Terminator : Terminator
  Fxyz Mxyz : Outport
  wires:
  Mux/1 -> Fxyz Mxyz/1
  Constant1/1 -> "Aerodynamic Forces and Moments "/4
  Coef/1 -> "Aerodynamic Forces and Moments "/1
  Constant/1 -> "Aerodynamic Forces and Moments "/3
  "Aerodynamic Forces and Moments "/1 -> Mux/1
  "Aerodynamic Forces and Moments "/2 -> Mux/2
  Dynamic Pressure [Pa]/1 -> "Aerodynamic Forces and Moments "/2
  Body Velocity [m/s]/1 -> Terminator/1

== system uas_sim/Vehicle/Forces and Moments/Aerodynamic/Aerodynamic Forces and Moments Coef Axis Variant/Stability Axis Coef ==
  Coef : Inport
  Dynamic Pressure [Pa] : Inport  Port=2
  Body Velocity [m/s] : Inport  Port=3
  "Aerodynamic Forces and Moments " : aerolibadyn/Aerodynamic Forces and Moments   inputAxes=Stability  outputForceAxes=Body  outputMomentAxes=Body  S=Aircraft.Geom.s_m2  b=Aircraft.Geom.b_m  cbar=Aircraft.Geom.c_m
  Constant : Constant  Value=Aircraft.Mass.cg_m
  Constant1 : Constant  Value=Aircraft.Geom.cp_m
  Mux : Mux  Inputs=2
  Fxyz Mxyz : Outport
  wires:
  Dynamic Pressure [Pa]/1 -> "Aerodynamic Forces and Moments "/2
  "Aerodynamic Forces and Moments "/2 -> Mux/2
  "Aerodynamic Forces and Moments "/1 -> Mux/1
  Constant/1 -> "Aerodynamic Forces and Moments "/3
  Coef/1 -> "Aerodynamic Forces and Moments "/1
  Constant1/1 -> "Aerodynamic Forces and Moments "/4
  Mux/1 -> Fxyz Mxyz/1
  Body Velocity [m/s]/1 -> "Aerodynamic Forces and Moments "/5

== system uas_sim/Vehicle/Forces and Moments/Aerodynamic/Aerodynamic Forces and Moments Coef Axis Variant/Wind Axis Coef ==
  Coef : Inport
  Dynamic Pressure [Pa] : Inport  Port=2
  Body Velocity [m/s] : Inport  Port=3
  "Aerodynamic Forces and Moments " : aerolibadyn/Aerodynamic Forces and Moments   inputAxes=Wind  outputForceAxes=Body  outputMomentAxes=Body  S=Aircraft.Geom.s_m2  b=Aircraft.Geom.b_m  cbar=Aircraft.Geom.c_m
  Constant : Constant  Value=Aircraft.Mass.cg_m
  Constant1 : Constant  Value=Aircraft.Geom.cp_m
  Mux : Mux  Inputs=2
  Fxyz Mxyz : Outport
  wires:
  Dynamic Pressure [Pa]/1 -> "Aerodynamic Forces and Moments "/2
  Body Velocity [m/s]/1 -> "Aerodynamic Forces and Moments "/5
  "Aerodynamic Forces and Moments "/2 -> Mux/2
  "Aerodynamic Forces and Moments "/1 -> Mux/1
  Constant/1 -> "Aerodynamic Forces and Moments "/3
  Coef/1 -> "Aerodynamic Forces and Moments "/1
  Constant1/1 -> "Aerodynamic Forces and Moments "/4
  Mux/1 -> Fxyz Mxyz/1

== system uas_sim/Vehicle/Forces and Moments/Aerodynamic/Dynamic Derivatives/Pitch Rate ==
  Angle of Attack [rad] : Inport
  q_hat : Inport  Port=2
  CX q : Polyval  Coefs=Aircraft.Aero.CX.q
  CZ q : Polyval  Coefs=Aircraft.Aero.CZ.q
  Cm q : Polyval  Coefs=Aircraft.Aero.Cm.q
  Constant1 : Constant  Value=0
  Constant2 : Constant  Value=0
  Constant4 : Constant  Value=0
  Mux : Mux  Inputs=6
  Product : Product
  Product1 : Product
  Product2 : Product
  dC6 : Outport
  wires:
  Mux/1 -> dC6/1
  Constant1/1 -> Mux/2
  Product2/1 -> Mux/1
  Constant4/1 -> Mux/6
  Constant2/1 -> Mux/4
  Product/1 -> Mux/3
  Product1/1 -> Mux/5
  q_hat/1 -> Product2/2, Product1/2, Product/2
  CZ q/1 -> Product/1
  CX q/1 -> Product2/1
  Cm q/1 -> Product1/1
  Angle of Attack [rad]/1 -> CX q/1, Cm q/1, CZ q/1

== system uas_sim/Vehicle/Forces and Moments/Aerodynamic/Dynamic Derivatives/Roll Rate ==
  Angle of Attack [rad] : Inport
  p_hat : Inport  Port=2
  CY p : Polyval  Coefs=Aircraft.Aero.CY.p
  Cl p : Polyval  Coefs=Aircraft.Aero.Cl.p
  Cn p : Polyval  Coefs=Aircraft.Aero.Cn.p
  Constant : Constant  Value=0
  Constant2 : Constant  Value=0
  Constant4 : Constant  Value=0
  Mux : Mux  Inputs=6
  Product : Product
  Product1 : Product
  Product2 : Product
  dC6 : Outport
  wires:
  Product1/1 -> Mux/4
  Product2/1 -> Mux/6
  Constant/1 -> Mux/1
  Mux/1 -> dC6/1
  Product/1 -> Mux/2
  CY p/1 -> Product/1
  Cl p/1 -> Product1/1
  Constant2/1 -> Mux/3
  Constant4/1 -> Mux/5
  p_hat/1 -> Product2/2, Product1/2, Product/2
  Cn p/1 -> Product2/1
  Angle of Attack [rad]/1 -> Cn p/1, CY p/1, Cl p/1

== system uas_sim/Vehicle/Forces and Moments/Aerodynamic/Dynamic Derivatives/Yaw Rate ==
  Angle of Attack [rad] : Inport
  r_hat : Inport  Port=2
  CY r : Polyval  Coefs=Aircraft.Aero.CY.r
  Cl r : Polyval  Coefs=Aircraft.Aero.Cl.r
  Cn r : Polyval  Coefs=Aircraft.Aero.Cn.r
  Constant : Constant  Value=0
  Constant2 : Constant  Value=0
  Constant4 : Constant  Value=0
  Mux : Mux  Inputs=6
  Product : Product
  Product1 : Product
  Product2 : Product
  dC6 : Outport
  wires:
  r_hat/1 -> Product2/2, Product1/2, Product/2
  Mux/1 -> dC6/1
  CY r/1 -> Product/1
  Constant/1 -> Mux/1
  Product2/1 -> Mux/6
  Product/1 -> Mux/2
  Cl r/1 -> Product1/1
  Constant2/1 -> Mux/3
  Product1/1 -> Mux/4
  Constant4/1 -> Mux/5
  Cn r/1 -> Product2/1
  Angle of Attack [rad]/1 -> Cn r/1, CY r/1, Cl r/1

== matlab function uas_sim/Vehicle/Vehicle Model/MATLAB Function ==
  data: ang input; ret output
function ret  = constrain360(ang)
%Constrain360 Converts a +/-180 value to a 0 - 360 value
ret = fmod(ang, 360);
if ret < 0
    ret = ret + 360;
end

end

== matlab function uas_sim/Flight Management Unit/Sensor Models/GNSS/Triggered Subsystem/MATLAB Function ==
  data: year input; month input; mday input; hour input; minute input; second input; gnss_week output; sim_clock input; gnss_tow output
function [gnss_week, gnss_tow] = GnssWeekAndTime(year, month, mday, hour, minute, second, sim_clock)

JAN61980 = 44244;
JAN11901 = 15385;
SEC_PER_DAY = 86400.0;

month_day = [
    0, 31, 59, 90, 120, 151, 181, 212, 243, 273, 304, 334;
    0, 31, 60, 91, 121, 152, 182, 213, 244, 274, 305, 335
];

second = second + sim_clock;
leap = (mod(year,4) == 0);
yday = month_day(leap + 1, month) + mday;
mjd = ((year - 1901) / 4) * 1461 + mod((year - 1901), 4) * 365 + yday - 1 + JAN11901;
fmjd = ((second / 60.0 + minute) / 60.0 + hour) / 24.0;
gnss_week = floor((mjd - JAN61980) / 7);
gnss_tow = ((mjd - JAN61980) - gnss_week * 7 + fmjd) * SEC_PER_DAY;

== matlab function uas_sim/Flight Management Unit/Sensor Models/GNSS/Triggered Subsystem/MATLAB Function1 ==
  data: ang input; ret output
function ret  = constrain360(ang)
%Constrain360 Converts a +/-180 value to a 0 - 360 value
ret = fmod(ang, 360);
if ret < 0
    ret = ret + 360;
end

end
